simulink model "SMC_ThreeLink"  (R2020b)
settings: Solver=VariableStepAuto  StartTime=0.0  StopTime=20  RelTol=1e-3
settings Model: Creator=MR.co  LastModifiedBy=Taha

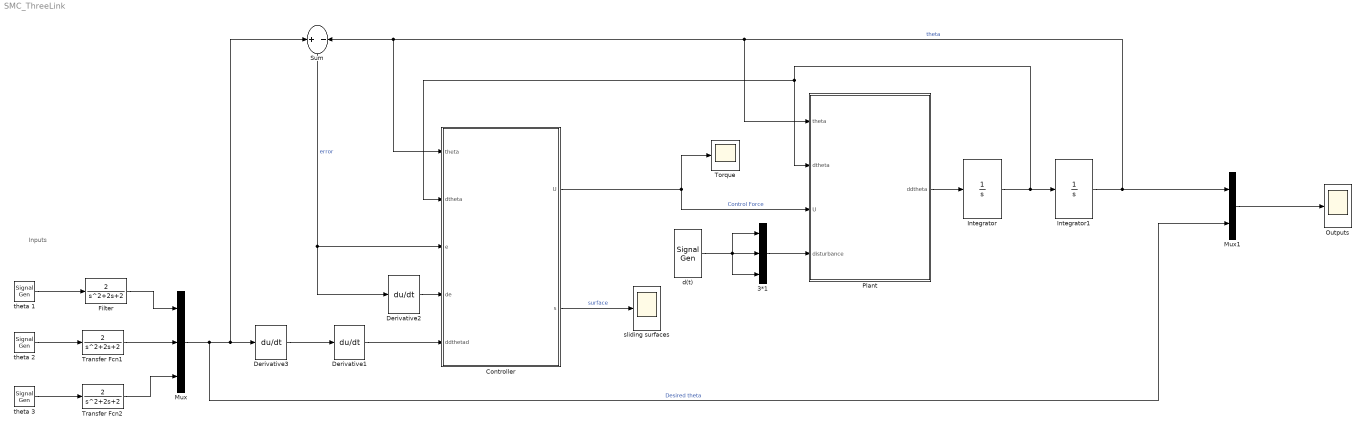
== system SMC_ThreeLink ==
  note: Inputs
  3*1 : Mux  Inputs=3
  Controller : MATLAB Function  TreatAsAtomicUnit=on
  Derivative1 : Derivative
  Derivative2 : Derivative
  Derivative3 : Derivative
  Filter : TransferFcn  Numerator=[2]  Denominator=[1 2 2]
  Integrator : Integrator  InitialCondition=randn(3,1)
  Integrator1 : Integrator  InitialCondition=randn(3,1)
  Mux : Mux  Inputs=3
  Mux1 : Mux  Inputs=2
  Outputs : Scope
  Plant : MATLAB Function  TreatAsAtomicUnit=on
  Sum : Sum  Inputs=+|-
  Torque : Scope
  Transfer Fcn1 : TransferFcn  Numerator=[2]  Denominator=[1 2 2]
  Transfer Fcn2 : TransferFcn  Numerator=[2]  Denominator=[1 2 2]
  d(t) : SignalGenerator  Amplitude=10  Frequency=pi  Units=rad/sec
  sliding surfaces : Scope
  theta 1 : SignalGenerator  Amplitude=2  Frequency=pi  Units=rad/sec
  theta 2 : SignalGenerator  WaveForm=square  Amplitude=3  Frequency=pi/2  Units=rad/sec
  theta 3 : SignalGenerator  WaveForm=square  Frequency=pi/3  Units=rad/sec
  wires:
  theta 1/1 -> Filter/1
  Mux/1 -> Derivative3/1, Sum/1, Mux1/2  "Desired theta"
  Integrator1/1 -> Plant/1(theta), Controller/1(theta), Sum/2, Mux1/1  "theta"
  Derivative2/1 -> Controller/4(de)
  Controller/2(s) -> sliding surfaces/1  "surface"
  theta 2/1 -> Transfer Fcn1/1
  Filter/1 -> Mux/1
  Derivative1/1 -> Controller/5(ddthetad)
  Mux1/1 -> Outputs/1
  Integrator/1 -> Controller/2(dtheta), Plant/2(dtheta), Integrator1/1
  Controller/1(U) -> Torque/1, Plant/3(U)  "Control Force"
  Plant/1(ddtheta) -> Integrator/1
  Sum/1 -> Derivative2/1, Controller/3(e)  "error"
  Transfer Fcn1/1 -> Mux/2
  Transfer Fcn2/1 -> Mux/3
  theta 3/1 -> Transfer Fcn2/1
  d(t)/1 -> 3*1/1, 3*1/3, 3*1/2
  3*1/1 -> Plant/4(disturbance)
  Derivative3/1 -> Derivative1/1

== matlab function SMC_ThreeLink/Controller ==
  data: theta input; U output; dtheta input; e input; de input; ddthetad input; s output
function [U , s]= fcn( theta , dtheta , e , de, ddthetad)


    m1 = 1 ;                % mass of link1 (kg)
    m2 = 1 ;                % mass of link2 (kg)
    m3 = 1 ;                % mass of link3 (kg)

    a1 = 1 ;                 % Length of link1 (m)
    a2 = 1 ;                 % Length of link2 (m)
    a3 = 1 ;                 % Length of link3 (m)
    
    ac1 = a1 / 2 ;         % Center of mass 1 (m)
    ac2 = a2 / 2 ;         % Center of mass 2 (m)
    ac3 = a3 / 2 ;         % Center of mass 3 (m)


    I1 = 1/12 * m1 * a1^2 ;   % Intertia of link1 (kg.N)
    I2 = 1/12 * m2 * a2^2 ;   % Intertia of link2 (kg.N)
    I3 = 1/12 * m3 * a3^2 ;   % Intertia of link3 (kg.N)

    g = 9.80665; % Gravity (m/s^2)

    
    M = zeros(3,3) ;    % Inertia Matrix
    
    M(1,1) = I1+I2+I3+m1*ac1^2+m2*(a1^2+ac2^2+ 2*a1*ac2*cos(theta(2)))+m3*(a1^2+a2^2+ac3^2+2*a1*a2*cos(theta(2))+2*a1*ac3*cos(theta(2)+theta(3))+2*a2*ac3*cos(theta(3)) );
    M(1,2) = I2+I3 + m2*(ac2^2+a1*ac2*cos(theta(2)))+m3*(a2^2+ac3^2+a1*a2*cos(theta(2))+2*a2*ac3*cos(theta(3))+a1*ac3*cos(theta(2)+theta(3)) );
    M(2,1) = M(1,2) ;    
    M(3,1) = I3+m3*(ac3^2+a2*ac3*cos(theta(3))+a1*ac3*cos(theta(2)+theta(3)) );
    M(1,3) = M(3,1) ;
    M(3,2) = I3+m3*(ac3^2+a2*ac3*cos(theta(3))) ;
    M(2,3) = M(3,2) ;
    M(2,2) = I2+I3+m2*ac2^2+m3*((a2^2+ac3^2)+2*a2*ac3*cos(theta(3))) ;
    M(3,3) = I3+m3*ac3^2 ;

    B=zeros(3,1);

    B(1) = -m2*a1*ac2*(2*dtheta(1)+dtheta(2))*sin(theta(2))* dtheta(2)...
        -m3*(a1*a2*(2*dtheta(1)+dtheta(2))*sin(theta(2))+a1*ac3*(2*dtheta(1)+dtheta(2)+dtheta(3))*sin(theta(2)+theta(3))+a2*ac3*(2*dtheta(1)+dtheta(2)+dtheta(3))*sin(theta(3)));

    B(2) = -m2*(a1*ac2*((dtheta(1)^2)+dtheta(1)*dtheta(2))*sin(theta(2)) + a1*ac2*dtheta(1)*sin(theta(2))*dtheta(2))-...
        m3*(a1*a2*((dtheta(1)^2)+dtheta(1)*dtheta(2)) + a1*ac3*((dtheta(1)^2)+dtheta(1)*dtheta(2)+dtheta(1)*dtheta(3))*sin(theta(2)+theta(3)) + ...
        a2*ac3*((dtheta(1)^2)+2*dtheta(1)*dtheta(2)+dtheta(1)*dtheta(3)+(dtheta(2)^2)+dtheta(2)*dtheta(3))*sin(theta(3)) + ...
        a1*a2*dtheta(1)*sin(theta(2))*dtheta(2) + a1*ac3*dtheta(1)*dtheta(2)*sin(theta(2)+theta(3)) + ...
        a2*ac3*(2*dtheta(1)+2*dtheta(2)+dtheta(3))*sin(theta(3)));

    B(3) = -m3*(a1*ac3*((dtheta(1)^2)+dtheta(1)*dtheta(2)+dtheta(1)*dtheta(3))*sin(theta(2)+theta(3))+ ...
        a2*ac3*((dtheta(1)^2)+2*dtheta(1)*dtheta(2)+dtheta(1)*dtheta(3)+(dtheta(2)^2)+dtheta(2)*dtheta(3))*sin(theta(3)) + ...
        a1*ac3*dtheta(1)*dtheta(3)*sin(theta(2)+theta(3)) + ...
        a2*ac3*(dtheta(1)+dtheta(2))*sin(theta(3))*dtheta(3));

    G = zeros(3,1);  % Gravity Matrix

    G(1) = g * ( cos(theta(1)) * (m1 * ac1 + m2 * a1 + m3 * a1) + cos(theta(1)+theta(2)) * (m2 * ac2 + m3 * a2) + cos(theta(1) + theta(2) + theta(3)) * (m3 * ac3));
    G(2) = g * ((m2 * ac2 + m3 * a2) * cos(theta(1)+theta(2)) + m3 * ac3 * cos(theta(1) + theta(2) + theta(3)));
    G(3) = g *(m3 * ac3 * cos(theta(1) + theta(2) + theta(3)));

    % sdot = -alpha * s + beta * tanh(s)
    
    alpha = 10 * eye(3);
    beta = 10 * [8 0 0;0 10 0 ; 0 0 20];
        
    
    c =  10 * eye(3);
    s = de + c * e; 
    
    D = 8 * eye(3);
    
    U = M * (ddthetad + c* de + (beta + D)* tanh(s) + alpha*s) + B + G;

== matlab function SMC_ThreeLink/Plant ==
  data: theta input; ddtheta output; dtheta input; U input; disturbance input
function ddtheta = fcn( theta , dtheta , U , disturbance)


    m1 = 1 ; %kg
    m2 = 1 ; %kg
    m3 = 1 ; %kg

    ac1 = .5 ; %m
    ac2 = .5 ; %m
    ac3 = .5 ; %m

    a1 = 1 ; %m
    a2 = 1 ; %m
    a3 = 1 ; %m

    I1 = 1/12 * m1 * a1^2 ; %kg.N
    I2 = 1/12 * m2 * a2^2 ; %kg.N
    I3 = 1/12 * m3 * a3^2 ; %kg.N

    g = 9.8; %m/s^2


    M = zeros(3,3) ;
    M(1,1) = I1+I2+I3+m1*ac1^2+m2*(a1^2+ac2^2+ 2*a1*ac2*cos(theta(2)))+m3*(a1^2+a2^2+ac3^2+2*a1*a2*cos(theta(2))+2*a1*ac3*cos(theta(2)+theta(3))+2*a2*ac3*cos(theta(3)) );
    M(1,2) = I2+I3 + m2*(ac2^2+a1*ac2*cos(theta(2)))+m3*(a2^2+ac3^2+a1*a2*cos(theta(2))+2*a2*ac3*cos(theta(3))+a1*ac3*cos(theta(2)+theta(3)) );
    M(2,1) = M(1,2) ;    
    M(3,1) = I3+m3*(ac3^2+a2*ac3*cos(theta(3))+a1*ac3*cos(theta(2)+theta(3)) );
    M(1,3) = M(3,1) ;
    M(3,2) = I3+m3*(ac3^2+a2*ac3*cos(theta(3))) ;
    M(2,3) = M(3,2) ;
    M(2,2) = I2+I3+m2*ac2^2+m3*((a2^2+ac3^2)+2*a2*ac3*cos(theta(3))) ;
    M(3,3) = I3+m3*ac3^2 ;

    B=zeros(3,1);

    B(1) = -m2*a1*ac2*(2*dtheta(1)+dtheta(2))*sin(theta(2))* dtheta(2)...
        -m3*(a1*a2*(2*dtheta(1)+dtheta(2))*sin(theta(2))+a1*ac3*(2*dtheta(1)+dtheta(2)+dtheta(3))*sin(theta(2)+theta(3))+a2*ac3*(2*dtheta(1)+dtheta(2)+dtheta(3))*sin(theta(3)));

    B(2) = -m2*(a1*ac2*((dtheta(1)^2)+dtheta(1)*dtheta(2))*sin(theta(2)) + a1*ac2*dtheta(1)*sin(theta(2))*dtheta(2))-...
        m3*(a1*a2*((dtheta(1)^2)+dtheta(1)*dtheta(2)) + a1*ac3*((dtheta(1)^2)+dtheta(1)*dtheta(2)+dtheta(1)*dtheta(3))*sin(theta(2)+theta(3)) + ...
        a2*ac3*((dtheta(1)^2)+2*dtheta(1)*dtheta(2)+dtheta(1)*dtheta(3)+(dtheta(2)^2)+dtheta(2)*dtheta(3))*sin(theta(3)) + ...
        a1*a2*dtheta(1)*sin(theta(2))*dtheta(2) + a1*ac3*dtheta(1)*dtheta(2)*sin(theta(2)+theta(3)) + ...
        a2*ac3*(2*dtheta(1)+2*dtheta(2)+dtheta(3))*sin(theta(3)));

    B(3) = -m3*(a1*ac3*((dtheta(1)^2)+dtheta(1)*dtheta(2)+dtheta(1)*dtheta(3))*sin(theta(2)+theta(3))+ ...
        a2*ac3*((dtheta(1)^2)+2*dtheta(1)*dtheta(2)+dtheta(1)*dtheta(3)+(dtheta(2)^2)+dtheta(2)*dtheta(3))*sin(theta(3)) + ...
        a1*ac3*dtheta(1)*dtheta(3)*sin(theta(2)+theta(3)) + ...
        a2*ac3*(dtheta(1)+dtheta(2))*sin(theta(3))*dtheta(3));

    G = zeros(3,1);

    G(1) = g * ( cos(theta(1)) * (m1 * ac1 + m2 * a1 + m3 * a1) + cos(theta(1)+theta(2)) * (m2 * ac2 + m3 * a2) + cos(theta(1) + theta(2) + theta(3)) * (m3 * ac3));
    G(2) = g * ((m2 * ac2 + m3 * a2) * cos(theta(1)+theta(2)) + m3 * ac3 * cos(theta(1) + theta(2) + theta(3)));
    G(3) = g *(m3 * ac3 * cos(theta(1) + theta(2) + theta(3)));

    ddtheta = M\(U -B - G + disturbance) ;
